simulink model "R"  (R2024a)
settings: Solver=VariableStepAuto  StartTime=0.0  StopTime=10*10^-6  RelTol=1e-3
undefined symbols (not defined in the file): c1, c3, rxDpIndex
libraries: commblkcod2 x64, commofdm x64, commdigbbndam3 x64, commsink2 x1, commseqgen3 x1
(part 2 of 3)

== system R/4K QAM/MSC13 WiFi Modulation29 ==
  In1 : Inport
  BCH Encoder : commblkcod2/BCH Encoder  n=47040  k=39200  specShortening=off  shortenedK=5  specGenPoly=off  genPoly='X^10 + X^8 + X^5 + X^4 + X^2 + X + 1'  specPrimPoly=off  prPoly='X^4 + X + 1'  specDisableGenCheck=off  specPuncture=off  punctVec=[ones(8,1); zeros(2,1)]
  OFDM Modulator : commofdm/OFDM Modulator  StatePerturbationForJacobian=1.0e-05  FFTLength=4096  NumGuardBandCarriers=[88; 88]  InsertDCNull=off  PilotInputPort=off  PilotCarrierIndices=[52;104;156;208;260]  CyclicPrefixLength=0  Windowing=off  WindowLength=1  OversamplingFactor=1  NumSymbols=1  NumTransmitAntennas=1  SimulateUsing=Interpreted execution
  Rectangular QAM Modulator Baseband : commdigbbndam3/Rectangular QAM Modulator Baseband  M=4096  InType=Bit  Enc=Gray  Mapping=[0:15]  PowType=Min. distance between symbols  MinDist=2  AvgPow=1  PeakPow=1  Ph=0  outDtype=double  outWordLen=16  outUDDataType=sfix(16)  outFracLenMode=Best precision  outFracLen=15  outDataTypeStr=double  outLastDataTypeStr=double
  Out1 : Outport
  wires:
  Rectangular QAM Modulator Baseband/1 -> OFDM Modulator/1
  OFDM Modulator/1 -> Out1/1
  BCH Encoder/1 -> Rectangular QAM Modulator Baseband/1
  In1/1 -> BCH Encoder/1

== system R/4K QAM/MSC13 WiFi Modulation3 ==
  In1 : Inport
  BCH Encoder : commblkcod2/BCH Encoder  n=47040  k=39200  specShortening=off  shortenedK=5  specGenPoly=off  genPoly='X^10 + X^8 + X^5 + X^4 + X^2 + X + 1'  specPrimPoly=off  prPoly='X^4 + X + 1'  specDisableGenCheck=off  specPuncture=off  punctVec=[ones(8,1); zeros(2,1)]
  OFDM Modulator : commofdm/OFDM Modulator  StatePerturbationForJacobian=1.0e-05  FFTLength=4096  NumGuardBandCarriers=[88; 88]  InsertDCNull=off  PilotInputPort=off  PilotCarrierIndices=[52;104;156;208;260]  CyclicPrefixLength=0  Windowing=off  WindowLength=1  OversamplingFactor=1  NumSymbols=1  NumTransmitAntennas=1  SimulateUsing=Interpreted execution
  Rectangular QAM Modulator Baseband : commdigbbndam3/Rectangular QAM Modulator Baseband  M=4096  InType=Bit  Enc=Gray  Mapping=[0:15]  PowType=Min. distance between symbols  MinDist=2  AvgPow=1  PeakPow=1  Ph=0  outDtype=double  outWordLen=16  outUDDataType=sfix(16)  outFracLenMode=Best precision  outFracLen=15  outDataTypeStr=double  outLastDataTypeStr=double
  Out1 : Outport
  wires:
  Rectangular QAM Modulator Baseband/1 -> OFDM Modulator/1
  OFDM Modulator/1 -> Out1/1
  BCH Encoder/1 -> Rectangular QAM Modulator Baseband/1
  In1/1 -> BCH Encoder/1

== system R/4K QAM/MSC13 WiFi Modulation30 ==
  In1 : Inport
  BCH Encoder : commblkcod2/BCH Encoder  n=47040  k=39200  specShortening=off  shortenedK=5  specGenPoly=off  genPoly='X^10 + X^8 + X^5 + X^4 + X^2 + X + 1'  specPrimPoly=off  prPoly='X^4 + X + 1'  specDisableGenCheck=off  specPuncture=off  punctVec=[ones(8,1); zeros(2,1)]
  OFDM Modulator : commofdm/OFDM Modulator  StatePerturbationForJacobian=1.0e-05  FFTLength=4096  NumGuardBandCarriers=[88; 88]  InsertDCNull=off  PilotInputPort=off  PilotCarrierIndices=[52;104;156;208;260]  CyclicPrefixLength=0  Windowing=off  WindowLength=1  OversamplingFactor=1  NumSymbols=1  NumTransmitAntennas=1  SimulateUsing=Interpreted execution
  Rectangular QAM Modulator Baseband : commdigbbndam3/Rectangular QAM Modulator Baseband  M=4096  InType=Bit  Enc=Gray  Mapping=[0:15]  PowType=Min. distance between symbols  MinDist=2  AvgPow=1  PeakPow=1  Ph=0  outDtype=double  outWordLen=16  outUDDataType=sfix(16)  outFracLenMode=Best precision  outFracLen=15  outDataTypeStr=double  outLastDataTypeStr=double
  Out1 : Outport
  wires:
  Rectangular QAM Modulator Baseband/1 -> OFDM Modulator/1
  OFDM Modulator/1 -> Out1/1
  BCH Encoder/1 -> Rectangular QAM Modulator Baseband/1
  In1/1 -> BCH Encoder/1

== system R/4K QAM/MSC13 WiFi Modulation31 ==
  In1 : Inport
  BCH Encoder : commblkcod2/BCH Encoder  n=47040  k=39200  specShortening=off  shortenedK=5  specGenPoly=off  genPoly='X^10 + X^8 + X^5 + X^4 + X^2 + X + 1'  specPrimPoly=off  prPoly='X^4 + X + 1'  specDisableGenCheck=off  specPuncture=off  punctVec=[ones(8,1); zeros(2,1)]
  OFDM Modulator : commofdm/OFDM Modulator  StatePerturbationForJacobian=1.0e-05  FFTLength=4096  NumGuardBandCarriers=[88; 88]  InsertDCNull=off  PilotInputPort=off  PilotCarrierIndices=[52;104;156;208;260]  CyclicPrefixLength=0  Windowing=off  WindowLength=1  OversamplingFactor=1  NumSymbols=1  NumTransmitAntennas=1  SimulateUsing=Interpreted execution
  Rectangular QAM Modulator Baseband : commdigbbndam3/Rectangular QAM Modulator Baseband  M=4096  InType=Bit  Enc=Gray  Mapping=[0:15]  PowType=Min. distance between symbols  MinDist=2  AvgPow=1  PeakPow=1  Ph=0  outDtype=double  outWordLen=16  outUDDataType=sfix(16)  outFracLenMode=Best precision  outFracLen=15  outDataTypeStr=double  outLastDataTypeStr=double
  Out1 : Outport
  wires:
  Rectangular QAM Modulator Baseband/1 -> OFDM Modulator/1
  OFDM Modulator/1 -> Out1/1
  BCH Encoder/1 -> Rectangular QAM Modulator Baseband/1
  In1/1 -> BCH Encoder/1

== system R/4K QAM/MSC13 WiFi Modulation4 ==
  In1 : Inport
  BCH Encoder : commblkcod2/BCH Encoder  n=47040  k=39200  specShortening=off  shortenedK=5  specGenPoly=off  genPoly='X^10 + X^8 + X^5 + X^4 + X^2 + X + 1'  specPrimPoly=off  prPoly='X^4 + X + 1'  specDisableGenCheck=off  specPuncture=off  punctVec=[ones(8,1); zeros(2,1)]
  OFDM Modulator : commofdm/OFDM Modulator  StatePerturbationForJacobian=1.0e-05  FFTLength=4096  NumGuardBandCarriers=[88; 88]  InsertDCNull=off  PilotInputPort=off  PilotCarrierIndices=[52;104;156;208;260]  CyclicPrefixLength=0  Windowing=off  WindowLength=1  OversamplingFactor=1  NumSymbols=1  NumTransmitAntennas=1  SimulateUsing=Interpreted execution
  Rectangular QAM Modulator Baseband : commdigbbndam3/Rectangular QAM Modulator Baseband  M=4096  InType=Bit  Enc=Gray  Mapping=[0:15]  PowType=Min. distance between symbols  MinDist=2  AvgPow=1  PeakPow=1  Ph=0  outDtype=double  outWordLen=16  outUDDataType=sfix(16)  outFracLenMode=Best precision  outFracLen=15  outDataTypeStr=double  outLastDataTypeStr=double
  Out1 : Outport
  wires:
  Rectangular QAM Modulator Baseband/1 -> OFDM Modulator/1
  OFDM Modulator/1 -> Out1/1
  BCH Encoder/1 -> Rectangular QAM Modulator Baseband/1
  In1/1 -> BCH Encoder/1

== system R/4K QAM/MSC13 WiFi Modulation5 ==
  In1 : Inport
  BCH Encoder : commblkcod2/BCH Encoder  n=47040  k=39200  specShortening=off  shortenedK=5  specGenPoly=off  genPoly='X^10 + X^8 + X^5 + X^4 + X^2 + X + 1'  specPrimPoly=off  prPoly='X^4 + X + 1'  specDisableGenCheck=off  specPuncture=off  punctVec=[ones(8,1); zeros(2,1)]
  OFDM Modulator : commofdm/OFDM Modulator  StatePerturbationForJacobian=1.0e-05  FFTLength=4096  NumGuardBandCarriers=[88; 88]  InsertDCNull=off  PilotInputPort=off  PilotCarrierIndices=[52;104;156;208;260]  CyclicPrefixLength=0  Windowing=off  WindowLength=1  OversamplingFactor=1  NumSymbols=1  NumTransmitAntennas=1  SimulateUsing=Interpreted execution
  Rectangular QAM Modulator Baseband : commdigbbndam3/Rectangular QAM Modulator Baseband  M=4096  InType=Bit  Enc=Gray  Mapping=[0:15]  PowType=Min. distance between symbols  MinDist=2  AvgPow=1  PeakPow=1  Ph=0  outDtype=double  outWordLen=16  outUDDataType=sfix(16)  outFracLenMode=Best precision  outFracLen=15  outDataTypeStr=double  outLastDataTypeStr=double
  Out1 : Outport
  wires:
  Rectangular QAM Modulator Baseband/1 -> OFDM Modulator/1
  OFDM Modulator/1 -> Out1/1
  BCH Encoder/1 -> Rectangular QAM Modulator Baseband/1
  In1/1 -> BCH Encoder/1

== system R/4K QAM/MSC13 WiFi Modulation6 ==
  In1 : Inport
  BCH Encoder : commblkcod2/BCH Encoder  n=47040  k=39200  specShortening=off  shortenedK=5  specGenPoly=off  genPoly='X^10 + X^8 + X^5 + X^4 + X^2 + X + 1'  specPrimPoly=off  prPoly='X^4 + X + 1'  specDisableGenCheck=off  specPuncture=off  punctVec=[ones(8,1); zeros(2,1)]
  OFDM Modulator : commofdm/OFDM Modulator  StatePerturbationForJacobian=1.0e-05  FFTLength=4096  NumGuardBandCarriers=[88; 88]  InsertDCNull=off  PilotInputPort=off  PilotCarrierIndices=[52;104;156;208;260]  CyclicPrefixLength=0  Windowing=off  WindowLength=1  OversamplingFactor=1  NumSymbols=1  NumTransmitAntennas=1  SimulateUsing=Interpreted execution
  Rectangular QAM Modulator Baseband : commdigbbndam3/Rectangular QAM Modulator Baseband  M=4096  InType=Bit  Enc=Gray  Mapping=[0:15]  PowType=Min. distance between symbols  MinDist=2  AvgPow=1  PeakPow=1  Ph=0  outDtype=double  outWordLen=16  outUDDataType=sfix(16)  outFracLenMode=Best precision  outFracLen=15  outDataTypeStr=double  outLastDataTypeStr=double
  Out1 : Outport
  wires:
  Rectangular QAM Modulator Baseband/1 -> OFDM Modulator/1
  OFDM Modulator/1 -> Out1/1
  BCH Encoder/1 -> Rectangular QAM Modulator Baseband/1
  In1/1 -> BCH Encoder/1

== system R/4K QAM/MSC13 WiFi Modulation7 ==
  In1 : Inport
  BCH Encoder : commblkcod2/BCH Encoder  n=47040  k=39200  specShortening=off  shortenedK=5  specGenPoly=off  genPoly='X^10 + X^8 + X^5 + X^4 + X^2 + X + 1'  specPrimPoly=off  prPoly='X^4 + X + 1'  specDisableGenCheck=off  specPuncture=off  punctVec=[ones(8,1); zeros(2,1)]
  OFDM Modulator : commofdm/OFDM Modulator  StatePerturbationForJacobian=1.0e-05  FFTLength=4096  NumGuardBandCarriers=[88; 88]  InsertDCNull=off  PilotInputPort=off  PilotCarrierIndices=[52;104;156;208;260]  CyclicPrefixLength=0  Windowing=off  WindowLength=1  OversamplingFactor=1  NumSymbols=1  NumTransmitAntennas=1  SimulateUsing=Interpreted execution
  Rectangular QAM Modulator Baseband : commdigbbndam3/Rectangular QAM Modulator Baseband  M=4096  InType=Bit  Enc=Gray  Mapping=[0:15]  PowType=Min. distance between symbols  MinDist=2  AvgPow=1  PeakPow=1  Ph=0  outDtype=double  outWordLen=16  outUDDataType=sfix(16)  outFracLenMode=Best precision  outFracLen=15  outDataTypeStr=double  outLastDataTypeStr=double
  Out1 : Outport
  wires:
  Rectangular QAM Modulator Baseband/1 -> OFDM Modulator/1
  OFDM Modulator/1 -> Out1/1
  BCH Encoder/1 -> Rectangular QAM Modulator Baseband/1
  In1/1 -> BCH Encoder/1

== system R/4K QAM/MSC13 WiFi Modulation8 ==
  In1 : Inport
  BCH Encoder : commblkcod2/BCH Encoder  n=47040  k=39200  specShortening=off  shortenedK=5  specGenPoly=off  genPoly='X^10 + X^8 + X^5 + X^4 + X^2 + X + 1'  specPrimPoly=off  prPoly='X^4 + X + 1'  specDisableGenCheck=off  specPuncture=off  punctVec=[ones(8,1); zeros(2,1)]
  OFDM Modulator : commofdm/OFDM Modulator  StatePerturbationForJacobian=1.0e-05  FFTLength=4096  NumGuardBandCarriers=[88; 88]  InsertDCNull=off  PilotInputPort=off  PilotCarrierIndices=[52;104;156;208;260]  CyclicPrefixLength=0  Windowing=off  WindowLength=1  OversamplingFactor=1  NumSymbols=1  NumTransmitAntennas=1  SimulateUsing=Interpreted execution
  Rectangular QAM Modulator Baseband : commdigbbndam3/Rectangular QAM Modulator Baseband  M=4096  InType=Bit  Enc=Gray  Mapping=[0:15]  PowType=Min. distance between symbols  MinDist=2  AvgPow=1  PeakPow=1  Ph=0  outDtype=double  outWordLen=16  outUDDataType=sfix(16)  outFracLenMode=Best precision  outFracLen=15  outDataTypeStr=double  outLastDataTypeStr=double
  Out1 : Outport
  wires:
  Rectangular QAM Modulator Baseband/1 -> OFDM Modulator/1
  OFDM Modulator/1 -> Out1/1
  BCH Encoder/1 -> Rectangular QAM Modulator Baseband/1
  In1/1 -> BCH Encoder/1

== system R/4K QAM/MSC13 WiFi Modulation9 ==
  In1 : Inport
  BCH Encoder : commblkcod2/BCH Encoder  n=47040  k=39200  specShortening=off  shortenedK=5  specGenPoly=off  genPoly='X^10 + X^8 + X^5 + X^4 + X^2 + X + 1'  specPrimPoly=off  prPoly='X^4 + X + 1'  specDisableGenCheck=off  specPuncture=off  punctVec=[ones(8,1); zeros(2,1)]
  OFDM Modulator : commofdm/OFDM Modulator  StatePerturbationForJacobian=1.0e-05  FFTLength=4096  NumGuardBandCarriers=[88; 88]  InsertDCNull=off  PilotInputPort=off  PilotCarrierIndices=[52;104;156;208;260]  CyclicPrefixLength=0  Windowing=off  WindowLength=1  OversamplingFactor=1  NumSymbols=1  NumTransmitAntennas=1  SimulateUsing=Interpreted execution
  Rectangular QAM Modulator Baseband : commdigbbndam3/Rectangular QAM Modulator Baseband  M=4096  InType=Bit  Enc=Gray  Mapping=[0:15]  PowType=Min. distance between symbols  MinDist=2  AvgPow=1  PeakPow=1  Ph=0  outDtype=double  outWordLen=16  outUDDataType=sfix(16)  outFracLenMode=Best precision  outFracLen=15  outDataTypeStr=double  outLastDataTypeStr=double
  Out1 : Outport
  wires:
  Rectangular QAM Modulator Baseband/1 -> OFDM Modulator/1
  OFDM Modulator/1 -> Out1/1
  BCH Encoder/1 -> Rectangular QAM Modulator Baseband/1
  In1/1 -> BCH Encoder/1

== system R/Subsystem1/MCS13 WiFi Demodulator1 ==
  In1 : Inport
  BCH Decoder1 : commblkcod2/BCH Decoder  n=47040  k=39200  specShortening=off  shortenedK=5  specGenPoly=off  genPoly='X^10 + X^8 + X^5 + X^4 + X^2 + X + 1'  specPrimPoly=off  prPoly='X^4 + X + 1'  specDisableGenCheck=off  specPuncture=off  punctVec=[ones(8,1); zeros(2,1)]  specErasurePort=off  showNumErr=off
  OFDM Demodulator1 : commofdm/OFDM Demodulator  StatePerturbationForJacobian=1.0e-05  FFTLength=4096  NumGuardBandCarriers=[88; 88]  RemoveDCCarrier=off  PilotOutputPort=off  PilotCarrierIndices=[35;60;85;110;135;160;185;210;235;260;285;310;335;360;385;410;435;460;485;510;535;560;585;610;635;660;685;710;735;760;785;810;835;860;885;910;935;960;985;1010;1035;1060;1085;1110;1135;1160;1185;1210;1235;1260;1285;1310;1335;1360;1385;1410;1435;1460;1485;1510;1535;1560;1585;1610;1635;1660;1685;1710;1735;1760;1785;1810;1835;1860;1885;1910;1935;1960;1985;2010;2035]  CyclicPrefixLength=0  OversamplingFactor=1  NumSymbols=1  NumReceiveAntennas=1  SimulateUsing=Interpreted execution
  Rectangular QAM Demodulator Baseband1 : commdigbbndam3/Rectangular QAM Demodulator Baseband  M=4096  OutType=Bit  DecType=Hard decision  VarSource=Dialog  Variance=1  Dec=Gray  Mapping=[0:15]  PowType=Min. distance between symbols  MinDist=2  AvgPow=1  PeakPow=1  Ph=0  outDtype1=Inherit via internal rule  outDtype2=Inherit via internal rule  derotateFactorWordLen=16  derotateFactorDataTypeStr=Inherit: Same word length as input  derotateFactorLastDataTypeStr=Inherit: Same word length as input  denormFactorWordLen=16  denormFactorDataTypeStr=Inherit: Same word length as input  denormFactorLastDataTypeStr=Inherit: Same word length as input  prodOutWordLen=32  prodOutOverflowMode=Wrap  prodOutRoundingMode=Floor  prodOutOvFlMode=off  prodOutOvFlModeLastStrValue=off  sumWordLen=32
      settings: LibrarySourceBlock=|
      | commhdldigbbndam/Rectangular QAM
      | Demodulator
      | Baseband
  Out1 : Outport
  wires:
  BCH Decoder1/1 -> Out1/1
  OFDM Demodulator1/1 -> Rectangular QAM Demodulator Baseband1/1
  In1/1 -> OFDM Demodulator1/1
  Rectangular QAM Demodulator Baseband1/1 -> BCH Decoder1/1

== system R/Subsystem1/MCS13 WiFi Demodulator10 ==
  In1 : Inport
  BCH Decoder1 : commblkcod2/BCH Decoder  n=47040  k=39200  specShortening=off  shortenedK=5  specGenPoly=off  genPoly='X^10 + X^8 + X^5 + X^4 + X^2 + X + 1'  specPrimPoly=off  prPoly='X^4 + X + 1'  specDisableGenCheck=off  specPuncture=off  punctVec=[ones(8,1); zeros(2,1)]  specErasurePort=off  showNumErr=off
  OFDM Demodulator1 : commofdm/OFDM Demodulator  StatePerturbationForJacobian=1.0e-05  FFTLength=4096  NumGuardBandCarriers=[88; 88]  RemoveDCCarrier=off  PilotOutputPort=off  PilotCarrierIndices=[35;60;85;110;135;160;185;210;235;260;285;310;335;360;385;410;435;460;485;510;535;560;585;610;635;660;685;710;735;760;785;810;835;860;885;910;935;960;985;1010;1035;1060;1085;1110;1135;1160;1185;1210;1235;1260;1285;1310;1335;1360;1385;1410;1435;1460;1485;1510;1535;1560;1585;1610;1635;1660;1685;1710;1735;1760;1785;1810;1835;1860;1885;1910;1935;1960;1985;2010;2035]  CyclicPrefixLength=0  OversamplingFactor=1  NumSymbols=1  NumReceiveAntennas=1  SimulateUsing=Interpreted execution
  Rectangular QAM Demodulator Baseband1 : commdigbbndam3/Rectangular QAM Demodulator Baseband  M=4096  OutType=Bit  DecType=Hard decision  VarSource=Dialog  Variance=1  Dec=Gray  Mapping=[0:15]  PowType=Min. distance between symbols  MinDist=2  AvgPow=1  PeakPow=1  Ph=0  outDtype1=Inherit via internal rule  outDtype2=Inherit via internal rule  derotateFactorWordLen=16  derotateFactorDataTypeStr=Inherit: Same word length as input  derotateFactorLastDataTypeStr=Inherit: Same word length as input  denormFactorWordLen=16  denormFactorDataTypeStr=Inherit: Same word length as input  denormFactorLastDataTypeStr=Inherit: Same word length as input  prodOutWordLen=32  prodOutOverflowMode=Wrap  prodOutRoundingMode=Floor  prodOutOvFlMode=off  prodOutOvFlModeLastStrValue=off  sumWordLen=32
      settings: LibrarySourceBlock=|
      | commhdldigbbndam/Rectangular QAM
      | Demodulator
      | Baseband
  Out1 : Outport
  wires:
  BCH Decoder1/1 -> Out1/1
  OFDM Demodulator1/1 -> Rectangular QAM Demodulator Baseband1/1
  In1/1 -> OFDM Demodulator1/1
  Rectangular QAM Demodulator Baseband1/1 -> BCH Decoder1/1

== system R/Subsystem1/MCS13 WiFi Demodulator11 ==
  In1 : Inport
  BCH Decoder1 : commblkcod2/BCH Decoder  n=47040  k=39200  specShortening=off  shortenedK=5  specGenPoly=off  genPoly='X^10 + X^8 + X^5 + X^4 + X^2 + X + 1'  specPrimPoly=off  prPoly='X^4 + X + 1'  specDisableGenCheck=off  specPuncture=off  punctVec=[ones(8,1); zeros(2,1)]  specErasurePort=off  showNumErr=off
  OFDM Demodulator1 : commofdm/OFDM Demodulator  StatePerturbationForJacobian=1.0e-05  FFTLength=4096  NumGuardBandCarriers=[88; 88]  RemoveDCCarrier=off  PilotOutputPort=off  PilotCarrierIndices=[35;60;85;110;135;160;185;210;235;260;285;310;335;360;385;410;435;460;485;510;535;560;585;610;635;660;685;710;735;760;785;810;835;860;885;910;935;960;985;1010;1035;1060;1085;1110;1135;1160;1185;1210;1235;1260;1285;1310;1335;1360;1385;1410;1435;1460;1485;1510;1535;1560;1585;1610;1635;1660;1685;1710;1735;1760;1785;1810;1835;1860;1885;1910;1935;1960;1985;2010;2035]  CyclicPrefixLength=0  OversamplingFactor=1  NumSymbols=1  NumReceiveAntennas=1  SimulateUsing=Interpreted execution
  Rectangular QAM Demodulator Baseband1 : commdigbbndam3/Rectangular QAM Demodulator Baseband  M=4096  OutType=Bit  DecType=Hard decision  VarSource=Dialog  Variance=1  Dec=Gray  Mapping=[0:15]  PowType=Min. distance between symbols  MinDist=2  AvgPow=1  PeakPow=1  Ph=0  outDtype1=Inherit via internal rule  outDtype2=Inherit via internal rule  derotateFactorWordLen=16  derotateFactorDataTypeStr=Inherit: Same word length as input  derotateFactorLastDataTypeStr=Inherit: Same word length as input  denormFactorWordLen=16  denormFactorDataTypeStr=Inherit: Same word length as input  denormFactorLastDataTypeStr=Inherit: Same word length as input  prodOutWordLen=32  prodOutOverflowMode=Wrap  prodOutRoundingMode=Floor  prodOutOvFlMode=off  prodOutOvFlModeLastStrValue=off  sumWordLen=32
      settings: LibrarySourceBlock=|
      | commhdldigbbndam/Rectangular QAM
      | Demodulator
      | Baseband
  Out1 : Outport
  wires:
  BCH Decoder1/1 -> Out1/1
  OFDM Demodulator1/1 -> Rectangular QAM Demodulator Baseband1/1
  In1/1 -> OFDM Demodulator1/1
  Rectangular QAM Demodulator Baseband1/1 -> BCH Decoder1/1

== system R/Subsystem1/MCS13 WiFi Demodulator12 ==
  In1 : Inport
  BCH Decoder1 : commblkcod2/BCH Decoder  n=47040  k=39200  specShortening=off  shortenedK=5  specGenPoly=off  genPoly='X^10 + X^8 + X^5 + X^4 + X^2 + X + 1'  specPrimPoly=off  prPoly='X^4 + X + 1'  specDisableGenCheck=off  specPuncture=off  punctVec=[ones(8,1); zeros(2,1)]  specErasurePort=off  showNumErr=off
  OFDM Demodulator1 : commofdm/OFDM Demodulator  StatePerturbationForJacobian=1.0e-05  FFTLength=4096  NumGuardBandCarriers=[88; 88]  RemoveDCCarrier=off  PilotOutputPort=off  PilotCarrierIndices=[35;60;85;110;135;160;185;210;235;260;285;310;335;360;385;410;435;460;485;510;535;560;585;610;635;660;685;710;735;760;785;810;835;860;885;910;935;960;985;1010;1035;1060;1085;1110;1135;1160;1185;1210;1235;1260;1285;1310;1335;1360;1385;1410;1435;1460;1485;1510;1535;1560;1585;1610;1635;1660;1685;1710;1735;1760;1785;1810;1835;1860;1885;1910;1935;1960;1985;2010;2035]  CyclicPrefixLength=0  OversamplingFactor=1  NumSymbols=1  NumReceiveAntennas=1  SimulateUsing=Interpreted execution
  Rectangular QAM Demodulator Baseband1 : commdigbbndam3/Rectangular QAM Demodulator Baseband  M=4096  OutType=Bit  DecType=Hard decision  VarSource=Dialog  Variance=1  Dec=Gray  Mapping=[0:15]  PowType=Min. distance between symbols  MinDist=2  AvgPow=1  PeakPow=1  Ph=0  outDtype1=Inherit via internal rule  outDtype2=Inherit via internal rule  derotateFactorWordLen=16  derotateFactorDataTypeStr=Inherit: Same word length as input  derotateFactorLastDataTypeStr=Inherit: Same word length as input  denormFactorWordLen=16  denormFactorDataTypeStr=Inherit: Same word length as input  denormFactorLastDataTypeStr=Inherit: Same word length as input  prodOutWordLen=32  prodOutOverflowMode=Wrap  prodOutRoundingMode=Floor  prodOutOvFlMode=off  prodOutOvFlModeLastStrValue=off  sumWordLen=32
      settings: LibrarySourceBlock=|
      | commhdldigbbndam/Rectangular QAM
      | Demodulator
      | Baseband
  Out1 : Outport
  wires:
  BCH Decoder1/1 -> Out1/1
  OFDM Demodulator1/1 -> Rectangular QAM Demodulator Baseband1/1
  In1/1 -> OFDM Demodulator1/1
  Rectangular QAM Demodulator Baseband1/1 -> BCH Decoder1/1

== system R/Subsystem1/MCS13 WiFi Demodulator13 ==
  In1 : Inport
  BCH Decoder1 : commblkcod2/BCH Decoder  n=47040  k=39200  specShortening=off  shortenedK=5  specGenPoly=off  genPoly='X^10 + X^8 + X^5 + X^4 + X^2 + X + 1'  specPrimPoly=off  prPoly='X^4 + X + 1'  specDisableGenCheck=off  specPuncture=off  punctVec=[ones(8,1); zeros(2,1)]  specErasurePort=off  showNumErr=off
  OFDM Demodulator1 : commofdm/OFDM Demodulator  StatePerturbationForJacobian=1.0e-05  FFTLength=4096  NumGuardBandCarriers=[88; 88]  RemoveDCCarrier=off  PilotOutputPort=off  PilotCarrierIndices=[35;60;85;110;135;160;185;210;235;260;285;310;335;360;385;410;435;460;485;510;535;560;585;610;635;660;685;710;735;760;785;810;835;860;885;910;935;960;985;1010;1035;1060;1085;1110;1135;1160;1185;1210;1235;1260;1285;1310;1335;1360;1385;1410;1435;1460;1485;1510;1535;1560;1585;1610;1635;1660;1685;1710;1735;1760;1785;1810;1835;1860;1885;1910;1935;1960;1985;2010;2035]  CyclicPrefixLength=0  OversamplingFactor=1  NumSymbols=1  NumReceiveAntennas=1  SimulateUsing=Interpreted execution
  Rectangular QAM Demodulator Baseband1 : commdigbbndam3/Rectangular QAM Demodulator Baseband  M=4096  OutType=Bit  DecType=Hard decision  VarSource=Dialog  Variance=1  Dec=Gray  Mapping=[0:15]  PowType=Min. distance between symbols  MinDist=2  AvgPow=1  PeakPow=1  Ph=0  outDtype1=Inherit via internal rule  outDtype2=Inherit via internal rule  derotateFactorWordLen=16  derotateFactorDataTypeStr=Inherit: Same word length as input  derotateFactorLastDataTypeStr=Inherit: Same word length as input  denormFactorWordLen=16  denormFactorDataTypeStr=Inherit: Same word length as input  denormFactorLastDataTypeStr=Inherit: Same word length as input  prodOutWordLen=32  prodOutOverflowMode=Wrap  prodOutRoundingMode=Floor  prodOutOvFlMode=off  prodOutOvFlModeLastStrValue=off  sumWordLen=32
      settings: LibrarySourceBlock=|
      | commhdldigbbndam/Rectangular QAM
      | Demodulator
      | Baseband
  Out1 : Outport
  wires:
  BCH Decoder1/1 -> Out1/1
  OFDM Demodulator1/1 -> Rectangular QAM Demodulator Baseband1/1
  In1/1 -> OFDM Demodulator1/1
  Rectangular QAM Demodulator Baseband1/1 -> BCH Decoder1/1

== system R/Subsystem1/MCS13 WiFi Demodulator14 ==
  In1 : Inport
  BCH Decoder1 : commblkcod2/BCH Decoder  n=47040  k=39200  specShortening=off  shortenedK=5  specGenPoly=off  genPoly='X^10 + X^8 + X^5 + X^4 + X^2 + X + 1'  specPrimPoly=off  prPoly='X^4 + X + 1'  specDisableGenCheck=off  specPuncture=off  punctVec=[ones(8,1); zeros(2,1)]  specErasurePort=off  showNumErr=off
  OFDM Demodulator1 : commofdm/OFDM Demodulator  StatePerturbationForJacobian=1.0e-05  FFTLength=4096  NumGuardBandCarriers=[88; 88]  RemoveDCCarrier=off  PilotOutputPort=off  PilotCarrierIndices=[35;60;85;110;135;160;185;210;235;260;285;310;335;360;385;410;435;460;485;510;535;560;585;610;635;660;685;710;735;760;785;810;835;860;885;910;935;960;985;1010;1035;1060;1085;1110;1135;1160;1185;1210;1235;1260;1285;1310;1335;1360;1385;1410;1435;1460;1485;1510;1535;1560;1585;1610;1635;1660;1685;1710;1735;1760;1785;1810;1835;1860;1885;1910;1935;1960;1985;2010;2035]  CyclicPrefixLength=0  OversamplingFactor=1  NumSymbols=1  NumReceiveAntennas=1  SimulateUsing=Interpreted execution
  Rectangular QAM Demodulator Baseband1 : commdigbbndam3/Rectangular QAM Demodulator Baseband  M=4096  OutType=Bit  DecType=Hard decision  VarSource=Dialog  Variance=1  Dec=Gray  Mapping=[0:15]  PowType=Min. distance between symbols  MinDist=2  AvgPow=1  PeakPow=1  Ph=0  outDtype1=Inherit via internal rule  outDtype2=Inherit via internal rule  derotateFactorWordLen=16  derotateFactorDataTypeStr=Inherit: Same word length as input  derotateFactorLastDataTypeStr=Inherit: Same word length as input  denormFactorWordLen=16  denormFactorDataTypeStr=Inherit: Same word length as input  denormFactorLastDataTypeStr=Inherit: Same word length as input  prodOutWordLen=32  prodOutOverflowMode=Wrap  prodOutRoundingMode=Floor  prodOutOvFlMode=off  prodOutOvFlModeLastStrValue=off  sumWordLen=32
      settings: LibrarySourceBlock=|
      | commhdldigbbndam/Rectangular QAM
      | Demodulator
      | Baseband
  Out1 : Outport
  wires:
  BCH Decoder1/1 -> Out1/1
  OFDM Demodulator1/1 -> Rectangular QAM Demodulator Baseband1/1
  In1/1 -> OFDM Demodulator1/1
  Rectangular QAM Demodulator Baseband1/1 -> BCH Decoder1/1

== system R/Subsystem1/MCS13 WiFi Demodulator15 ==
  In1 : Inport
  BCH Decoder1 : commblkcod2/BCH Decoder  n=47040  k=39200  specShortening=off  shortenedK=5  specGenPoly=off  genPoly='X^10 + X^8 + X^5 + X^4 + X^2 + X + 1'  specPrimPoly=off  prPoly='X^4 + X + 1'  specDisableGenCheck=off  specPuncture=off  punctVec=[ones(8,1); zeros(2,1)]  specErasurePort=off  showNumErr=off
  OFDM Demodulator1 : commofdm/OFDM Demodulator  StatePerturbationForJacobian=1.0e-05  FFTLength=4096  NumGuardBandCarriers=[88; 88]  RemoveDCCarrier=off  PilotOutputPort=off  PilotCarrierIndices=[35;60;85;110;135;160;185;210;235;260;285;310;335;360;385;410;435;460;485;510;535;560;585;610;635;660;685;710;735;760;785;810;835;860;885;910;935;960;985;1010;1035;1060;1085;1110;1135;1160;1185;1210;1235;1260;1285;1310;1335;1360;1385;1410;1435;1460;1485;1510;1535;1560;1585;1610;1635;1660;1685;1710;1735;1760;1785;1810;1835;1860;1885;1910;1935;1960;1985;2010;2035]  CyclicPrefixLength=0  OversamplingFactor=1  NumSymbols=1  NumReceiveAntennas=1  SimulateUsing=Interpreted execution
  Rectangular QAM Demodulator Baseband1 : commdigbbndam3/Rectangular QAM Demodulator Baseband  M=4096  OutType=Bit  DecType=Hard decision  VarSource=Dialog  Variance=1  Dec=Gray  Mapping=[0:15]  PowType=Min. distance between symbols  MinDist=2  AvgPow=1  PeakPow=1  Ph=0  outDtype1=Inherit via internal rule  outDtype2=Inherit via internal rule  derotateFactorWordLen=16  derotateFactorDataTypeStr=Inherit: Same word length as input  derotateFactorLastDataTypeStr=Inherit: Same word length as input  denormFactorWordLen=16  denormFactorDataTypeStr=Inherit: Same word length as input  denormFactorLastDataTypeStr=Inherit: Same word length as input  prodOutWordLen=32  prodOutOverflowMode=Wrap  prodOutRoundingMode=Floor  prodOutOvFlMode=off  prodOutOvFlModeLastStrValue=off  sumWordLen=32
      settings: LibrarySourceBlock=|
      | commhdldigbbndam/Rectangular QAM
      | Demodulator
      | Baseband
  Out1 : Outport
  wires:
  BCH Decoder1/1 -> Out1/1
  OFDM Demodulator1/1 -> Rectangular QAM Demodulator Baseband1/1
  In1/1 -> OFDM Demodulator1/1
  Rectangular QAM Demodulator Baseband1/1 -> BCH Decoder1/1

== system R/Subsystem1/MCS13 WiFi Demodulator16 ==
  In1 : Inport
  BCH Decoder1 : commblkcod2/BCH Decoder  n=47040  k=39200  specShortening=off  shortenedK=5  specGenPoly=off  genPoly='X^10 + X^8 + X^5 + X^4 + X^2 + X + 1'  specPrimPoly=off  prPoly='X^4 + X + 1'  specDisableGenCheck=off  specPuncture=off  punctVec=[ones(8,1); zeros(2,1)]  specErasurePort=off  showNumErr=off
  OFDM Demodulator1 : commofdm/OFDM Demodulator  StatePerturbationForJacobian=1.0e-05  FFTLength=4096  NumGuardBandCarriers=[88; 88]  RemoveDCCarrier=off  PilotOutputPort=off  PilotCarrierIndices=[35;60;85;110;135;160;185;210;235;260;285;310;335;360;385;410;435;460;485;510;535;560;585;610;635;660;685;710;735;760;785;810;835;860;885;910;935;960;985;1010;1035;1060;1085;1110;1135;1160;1185;1210;1235;1260;1285;1310;1335;1360;1385;1410;1435;1460;1485;1510;1535;1560;1585;1610;1635;1660;1685;1710;1735;1760;1785;1810;1835;1860;1885;1910;1935;1960;1985;2010;2035]  CyclicPrefixLength=0  OversamplingFactor=1  NumSymbols=1  NumReceiveAntennas=1  SimulateUsing=Interpreted execution
  Rectangular QAM Demodulator Baseband1 : commdigbbndam3/Rectangular QAM Demodulator Baseband  M=4096  OutType=Bit  DecType=Hard decision  VarSource=Dialog  Variance=1  Dec=Gray  Mapping=[0:15]  PowType=Min. distance between symbols  MinDist=2  AvgPow=1  PeakPow=1  Ph=0  outDtype1=Inherit via internal rule  outDtype2=Inherit via internal rule  derotateFactorWordLen=16  derotateFactorDataTypeStr=Inherit: Same word length as input  derotateFactorLastDataTypeStr=Inherit: Same word length as input  denormFactorWordLen=16  denormFactorDataTypeStr=Inherit: Same word length as input  denormFactorLastDataTypeStr=Inherit: Same word length as input  prodOutWordLen=32  prodOutOverflowMode=Wrap  prodOutRoundingMode=Floor  prodOutOvFlMode=off  prodOutOvFlModeLastStrValue=off  sumWordLen=32
      settings: LibrarySourceBlock=|
      | commhdldigbbndam/Rectangular QAM
      | Demodulator
      | Baseband
  Out1 : Outport
  wires:
  BCH Decoder1/1 -> Out1/1
  OFDM Demodulator1/1 -> Rectangular QAM Demodulator Baseband1/1
  In1/1 -> OFDM Demodulator1/1
  Rectangular QAM Demodulator Baseband1/1 -> BCH Decoder1/1

== system R/Subsystem1/MCS13 WiFi Demodulator17 ==
  In1 : Inport
  BCH Decoder1 : commblkcod2/BCH Decoder  n=47040  k=39200  specShortening=off  shortenedK=5  specGenPoly=off  genPoly='X^10 + X^8 + X^5 + X^4 + X^2 + X + 1'  specPrimPoly=off  prPoly='X^4 + X + 1'  specDisableGenCheck=off  specPuncture=off  punctVec=[ones(8,1); zeros(2,1)]  specErasurePort=off  showNumErr=off
  OFDM Demodulator1 : commofdm/OFDM Demodulator  StatePerturbationForJacobian=1.0e-05  FFTLength=4096  NumGuardBandCarriers=[88; 88]  RemoveDCCarrier=off  PilotOutputPort=off  PilotCarrierIndices=[35;60;85;110;135;160;185;210;235;260;285;310;335;360;385;410;435;460;485;510;535;560;585;610;635;660;685;710;735;760;785;810;835;860;885;910;935;960;985;1010;1035;1060;1085;1110;1135;1160;1185;1210;1235;1260;1285;1310;1335;1360;1385;1410;1435;1460;1485;1510;1535;1560;1585;1610;1635;1660;1685;1710;1735;1760;1785;1810;1835;1860;1885;1910;1935;1960;1985;2010;2035]  CyclicPrefixLength=0  OversamplingFactor=1  NumSymbols=1  NumReceiveAntennas=1  SimulateUsing=Interpreted execution
  Rectangular QAM Demodulator Baseband1 : commdigbbndam3/Rectangular QAM Demodulator Baseband  M=4096  OutType=Bit  DecType=Hard decision  VarSource=Dialog  Variance=1  Dec=Gray  Mapping=[0:15]  PowType=Min. distance between symbols  MinDist=2  AvgPow=1  PeakPow=1  Ph=0  outDtype1=Inherit via internal rule  outDtype2=Inherit via internal rule  derotateFactorWordLen=16  derotateFactorDataTypeStr=Inherit: Same word length as input  derotateFactorLastDataTypeStr=Inherit: Same word length as input  denormFactorWordLen=16  denormFactorDataTypeStr=Inherit: Same word length as input  denormFactorLastDataTypeStr=Inherit: Same word length as input  prodOutWordLen=32  prodOutOverflowMode=Wrap  prodOutRoundingMode=Floor  prodOutOvFlMode=off  prodOutOvFlModeLastStrValue=off  sumWordLen=32
      settings: LibrarySourceBlock=|
      | commhdldigbbndam/Rectangular QAM
      | Demodulator
      | Baseband
  Out1 : Outport
  wires:
  BCH Decoder1/1 -> Out1/1
  OFDM Demodulator1/1 -> Rectangular QAM Demodulator Baseband1/1
  In1/1 -> OFDM Demodulator1/1
  Rectangular QAM Demodulator Baseband1/1 -> BCH Decoder1/1

== system R/Subsystem1/MCS13 WiFi Demodulator18 ==
  In1 : Inport
  BCH Decoder1 : commblkcod2/BCH Decoder  n=47040  k=39200  specShortening=off  shortenedK=5  specGenPoly=off  genPoly='X^10 + X^8 + X^5 + X^4 + X^2 + X + 1'  specPrimPoly=off  prPoly='X^4 + X + 1'  specDisableGenCheck=off  specPuncture=off  punctVec=[ones(8,1); zeros(2,1)]  specErasurePort=off  showNumErr=off
  OFDM Demodulator1 : commofdm/OFDM Demodulator  StatePerturbationForJacobian=1.0e-05  FFTLength=4096  NumGuardBandCarriers=[88; 88]  RemoveDCCarrier=off  PilotOutputPort=off  PilotCarrierIndices=[35;60;85;110;135;160;185;210;235;260;285;310;335;360;385;410;435;460;485;510;535;560;585;610;635;660;685;710;735;760;785;810;835;860;885;910;935;960;985;1010;1035;1060;1085;1110;1135;1160;1185;1210;1235;1260;1285;1310;1335;1360;1385;1410;1435;1460;1485;1510;1535;1560;1585;1610;1635;1660;1685;1710;1735;1760;1785;1810;1835;1860;1885;1910;1935;1960;1985;2010;2035]  CyclicPrefixLength=0  OversamplingFactor=1  NumSymbols=1  NumReceiveAntennas=1  SimulateUsing=Interpreted execution
  Rectangular QAM Demodulator Baseband1 : commdigbbndam3/Rectangular QAM Demodulator Baseband  M=4096  OutType=Bit  DecType=Hard decision  VarSource=Dialog  Variance=1  Dec=Gray  Mapping=[0:15]  PowType=Min. distance between symbols  MinDist=2  AvgPow=1  PeakPow=1  Ph=0  outDtype1=Inherit via internal rule  outDtype2=Inherit via internal rule  derotateFactorWordLen=16  derotateFactorDataTypeStr=Inherit: Same word length as input  derotateFactorLastDataTypeStr=Inherit: Same word length as input  denormFactorWordLen=16  denormFactorDataTypeStr=Inherit: Same word length as input  denormFactorLastDataTypeStr=Inherit: Same word length as input  prodOutWordLen=32  prodOutOverflowMode=Wrap  prodOutRoundingMode=Floor  prodOutOvFlMode=off  prodOutOvFlModeLastStrValue=off  sumWordLen=32
      settings: LibrarySourceBlock=|
      | commhdldigbbndam/Rectangular QAM
      | Demodulator
      | Baseband
  Out1 : Outport
  wires:
  BCH Decoder1/1 -> Out1/1
  OFDM Demodulator1/1 -> Rectangular QAM Demodulator Baseband1/1
  In1/1 -> OFDM Demodulator1/1
  Rectangular QAM Demodulator Baseband1/1 -> BCH Decoder1/1

== system R/Subsystem1/MCS13 WiFi Demodulator19 ==
  In1 : Inport
  BCH Decoder1 : commblkcod2/BCH Decoder  n=47040  k=39200  specShortening=off  shortenedK=5  specGenPoly=off  genPoly='X^10 + X^8 + X^5 + X^4 + X^2 + X + 1'  specPrimPoly=off  prPoly='X^4 + X + 1'  specDisableGenCheck=off  specPuncture=off  punctVec=[ones(8,1); zeros(2,1)]  specErasurePort=off  showNumErr=off
  OFDM Demodulator1 : commofdm/OFDM Demodulator  StatePerturbationForJacobian=1.0e-05  FFTLength=4096  NumGuardBandCarriers=[88; 88]  RemoveDCCarrier=off  PilotOutputPort=off  PilotCarrierIndices=[35;60;85;110;135;160;185;210;235;260;285;310;335;360;385;410;435;460;485;510;535;560;585;610;635;660;685;710;735;760;785;810;835;860;885;910;935;960;985;1010;1035;1060;1085;1110;1135;1160;1185;1210;1235;1260;1285;1310;1335;1360;1385;1410;1435;1460;1485;1510;1535;1560;1585;1610;1635;1660;1685;1710;1735;1760;1785;1810;1835;1860;1885;1910;1935;1960;1985;2010;2035]  CyclicPrefixLength=0  OversamplingFactor=1  NumSymbols=1  NumReceiveAntennas=1  SimulateUsing=Interpreted execution
  Rectangular QAM Demodulator Baseband1 : commdigbbndam3/Rectangular QAM Demodulator Baseband  M=4096  OutType=Bit  DecType=Hard decision  VarSource=Dialog  Variance=1  Dec=Gray  Mapping=[0:15]  PowType=Min. distance between symbols  MinDist=2  AvgPow=1  PeakPow=1  Ph=0  outDtype1=Inherit via internal rule  outDtype2=Inherit via internal rule  derotateFactorWordLen=16  derotateFactorDataTypeStr=Inherit: Same word length as input  derotateFactorLastDataTypeStr=Inherit: Same word length as input  denormFactorWordLen=16  denormFactorDataTypeStr=Inherit: Same word length as input  denormFactorLastDataTypeStr=Inherit: Same word length as input  prodOutWordLen=32  prodOutOverflowMode=Wrap  prodOutRoundingMode=Floor  prodOutOvFlMode=off  prodOutOvFlModeLastStrValue=off  sumWordLen=32
      settings: LibrarySourceBlock=|
      | commhdldigbbndam/Rectangular QAM
      | Demodulator
      | Baseband
  Out1 : Outport
  wires:
  BCH Decoder1/1 -> Out1/1
  OFDM Demodulator1/1 -> Rectangular QAM Demodulator Baseband1/1
  In1/1 -> OFDM Demodulator1/1
  Rectangular QAM Demodulator Baseband1/1 -> BCH Decoder1/1

== system R/Subsystem1/MCS13 WiFi Demodulator2 ==
  In1 : Inport
  BCH Decoder1 : commblkcod2/BCH Decoder  n=47040  k=39200  specShortening=off  shortenedK=5  specGenPoly=off  genPoly='X^10 + X^8 + X^5 + X^4 + X^2 + X + 1'  specPrimPoly=off  prPoly='X^4 + X + 1'  specDisableGenCheck=off  specPuncture=off  punctVec=[ones(8,1); zeros(2,1)]  specErasurePort=off  showNumErr=off
  OFDM Demodulator1 : commofdm/OFDM Demodulator  StatePerturbationForJacobian=1.0e-05  FFTLength=4096  NumGuardBandCarriers=[88; 88]  RemoveDCCarrier=off  PilotOutputPort=off  PilotCarrierIndices=[35;60;85;110;135;160;185;210;235;260;285;310;335;360;385;410;435;460;485;510;535;560;585;610;635;660;685;710;735;760;785;810;835;860;885;910;935;960;985;1010;1035;1060;1085;1110;1135;1160;1185;1210;1235;1260;1285;1310;1335;1360;1385;1410;1435;1460;1485;1510;1535;1560;1585;1610;1635;1660;1685;1710;1735;1760;1785;1810;1835;1860;1885;1910;1935;1960;1985;2010;2035]  CyclicPrefixLength=0  OversamplingFactor=1  NumSymbols=1  NumReceiveAntennas=1  SimulateUsing=Interpreted execution
  Rectangular QAM Demodulator Baseband1 : commdigbbndam3/Rectangular QAM Demodulator Baseband  M=4096  OutType=Bit  DecType=Hard decision  VarSource=Dialog  Variance=1  Dec=Gray  Mapping=[0:15]  PowType=Min. distance between symbols  MinDist=2  AvgPow=1  PeakPow=1  Ph=0  outDtype1=Inherit via internal rule  outDtype2=Inherit via internal rule  derotateFactorWordLen=16  derotateFactorDataTypeStr=Inherit: Same word length as input  derotateFactorLastDataTypeStr=Inherit: Same word length as input  denormFactorWordLen=16  denormFactorDataTypeStr=Inherit: Same word length as input  denormFactorLastDataTypeStr=Inherit: Same word length as input  prodOutWordLen=32  prodOutOverflowMode=Wrap  prodOutRoundingMode=Floor  prodOutOvFlMode=off  prodOutOvFlModeLastStrValue=off  sumWordLen=32
      settings: LibrarySourceBlock=|
      | commhdldigbbndam/Rectangular QAM
      | Demodulator
      | Baseband
  Out1 : Outport
  wires:
  BCH Decoder1/1 -> Out1/1
  OFDM Demodulator1/1 -> Rectangular QAM Demodulator Baseband1/1
  In1/1 -> OFDM Demodulator1/1
  Rectangular QAM Demodulator Baseband1/1 -> BCH Decoder1/1

== system R/Subsystem1/MCS13 WiFi Demodulator20 ==
  In1 : Inport
  BCH Decoder1 : commblkcod2/BCH Decoder  n=47040  k=39200  specShortening=off  shortenedK=5  specGenPoly=off  genPoly='X^10 + X^8 + X^5 + X^4 + X^2 + X + 1'  specPrimPoly=off  prPoly='X^4 + X + 1'  specDisableGenCheck=off  specPuncture=off  punctVec=[ones(8,1); zeros(2,1)]  specErasurePort=off  showNumErr=off
  OFDM Demodulator1 : commofdm/OFDM Demodulator  StatePerturbationForJacobian=1.0e-05  FFTLength=4096  NumGuardBandCarriers=[88; 88]  RemoveDCCarrier=off  PilotOutputPort=off  PilotCarrierIndices=[35;60;85;110;135;160;185;210;235;260;285;310;335;360;385;410;435;460;485;510;535;560;585;610;635;660;685;710;735;760;785;810;835;860;885;910;935;960;985;1010;1035;1060;1085;1110;1135;1160;1185;1210;1235;1260;1285;1310;1335;1360;1385;1410;1435;1460;1485;1510;1535;1560;1585;1610;1635;1660;1685;1710;1735;1760;1785;1810;1835;1860;1885;1910;1935;1960;1985;2010;2035]  CyclicPrefixLength=0  OversamplingFactor=1  NumSymbols=1  NumReceiveAntennas=1  SimulateUsing=Interpreted execution
  Rectangular QAM Demodulator Baseband1 : commdigbbndam3/Rectangular QAM Demodulator Baseband  M=4096  OutType=Bit  DecType=Hard decision  VarSource=Dialog  Variance=1  Dec=Gray  Mapping=[0:15]  PowType=Min. distance between symbols  MinDist=2  AvgPow=1  PeakPow=1  Ph=0  outDtype1=Inherit via internal rule  outDtype2=Inherit via internal rule  derotateFactorWordLen=16  derotateFactorDataTypeStr=Inherit: Same word length as input  derotateFactorLastDataTypeStr=Inherit: Same word length as input  denormFactorWordLen=16  denormFactorDataTypeStr=Inherit: Same word length as input  denormFactorLastDataTypeStr=Inherit: Same word length as input  prodOutWordLen=32  prodOutOverflowMode=Wrap  prodOutRoundingMode=Floor  prodOutOvFlMode=off  prodOutOvFlModeLastStrValue=off  sumWordLen=32
      settings: LibrarySourceBlock=|
      | commhdldigbbndam/Rectangular QAM
      | Demodulator
      | Baseband
  Out1 : Outport
  wires:
  BCH Decoder1/1 -> Out1/1
  OFDM Demodulator1/1 -> Rectangular QAM Demodulator Baseband1/1
  In1/1 -> OFDM Demodulator1/1
  Rectangular QAM Demodulator Baseband1/1 -> BCH Decoder1/1

== system R/Subsystem1/MCS13 WiFi Demodulator21 ==
  In1 : Inport
  BCH Decoder1 : commblkcod2/BCH Decoder  n=47040  k=39200  specShortening=off  shortenedK=5  specGenPoly=off  genPoly='X^10 + X^8 + X^5 + X^4 + X^2 + X + 1'  specPrimPoly=off  prPoly='X^4 + X + 1'  specDisableGenCheck=off  specPuncture=off  punctVec=[ones(8,1); zeros(2,1)]  specErasurePort=off  showNumErr=off
  OFDM Demodulator1 : commofdm/OFDM Demodulator  StatePerturbationForJacobian=1.0e-05  FFTLength=4096  NumGuardBandCarriers=[88; 88]  RemoveDCCarrier=off  PilotOutputPort=off  PilotCarrierIndices=[35;60;85;110;135;160;185;210;235;260;285;310;335;360;385;410;435;460;485;510;535;560;585;610;635;660;685;710;735;760;785;810;835;860;885;910;935;960;985;1010;1035;1060;1085;1110;1135;1160;1185;1210;1235;1260;1285;1310;1335;1360;1385;1410;1435;1460;1485;1510;1535;1560;1585;1610;1635;1660;1685;1710;1735;1760;1785;1810;1835;1860;1885;1910;1935;1960;1985;2010;2035]  CyclicPrefixLength=0  OversamplingFactor=1  NumSymbols=1  NumReceiveAntennas=1  SimulateUsing=Interpreted execution
  Rectangular QAM Demodulator Baseband1 : commdigbbndam3/Rectangular QAM Demodulator Baseband  M=4096  OutType=Bit  DecType=Hard decision  VarSource=Dialog  Variance=1  Dec=Gray  Mapping=[0:15]  PowType=Min. distance between symbols  MinDist=2  AvgPow=1  PeakPow=1  Ph=0  outDtype1=Inherit via internal rule  outDtype2=Inherit via internal rule  derotateFactorWordLen=16  derotateFactorDataTypeStr=Inherit: Same word length as input  derotateFactorLastDataTypeStr=Inherit: Same word length as input  denormFactorWordLen=16  denormFactorDataTypeStr=Inherit: Same word length as input  denormFactorLastDataTypeStr=Inherit: Same word length as input  prodOutWordLen=32  prodOutOverflowMode=Wrap  prodOutRoundingMode=Floor  prodOutOvFlMode=off  prodOutOvFlModeLastStrValue=off  sumWordLen=32
      settings: LibrarySourceBlock=|
      | commhdldigbbndam/Rectangular QAM
      | Demodulator
      | Baseband
  Out1 : Outport
  wires:
  BCH Decoder1/1 -> Out1/1
  OFDM Demodulator1/1 -> Rectangular QAM Demodulator Baseband1/1
  In1/1 -> OFDM Demodulator1/1
  Rectangular QAM Demodulator Baseband1/1 -> BCH Decoder1/1

== system R/Subsystem1/MCS13 WiFi Demodulator22 ==
  In1 : Inport
  BCH Decoder1 : commblkcod2/BCH Decoder  n=47040  k=39200  specShortening=off  shortenedK=5  specGenPoly=off  genPoly='X^10 + X^8 + X^5 + X^4 + X^2 + X + 1'  specPrimPoly=off  prPoly='X^4 + X + 1'  specDisableGenCheck=off  specPuncture=off  punctVec=[ones(8,1); zeros(2,1)]  specErasurePort=off  showNumErr=off
  OFDM Demodulator1 : commofdm/OFDM Demodulator  StatePerturbationForJacobian=1.0e-05  FFTLength=4096  NumGuardBandCarriers=[88; 88]  RemoveDCCarrier=off  PilotOutputPort=off  PilotCarrierIndices=[35;60;85;110;135;160;185;210;235;260;285;310;335;360;385;410;435;460;485;510;535;560;585;610;635;660;685;710;735;760;785;810;835;860;885;910;935;960;985;1010;1035;1060;1085;1110;1135;1160;1185;1210;1235;1260;1285;1310;1335;1360;1385;1410;1435;1460;1485;1510;1535;1560;1585;1610;1635;1660;1685;1710;1735;1760;1785;1810;1835;1860;1885;1910;1935;1960;1985;2010;2035]  CyclicPrefixLength=0  OversamplingFactor=1  NumSymbols=1  NumReceiveAntennas=1  SimulateUsing=Interpreted execution
  Rectangular QAM Demodulator Baseband1 : commdigbbndam3/Rectangular QAM Demodulator Baseband  M=4096  OutType=Bit  DecType=Hard decision  VarSource=Dialog  Variance=1  Dec=Gray  Mapping=[0:15]  PowType=Min. distance between symbols  MinDist=2  AvgPow=1  PeakPow=1  Ph=0  outDtype1=Inherit via internal rule  outDtype2=Inherit via internal rule  derotateFactorWordLen=16  derotateFactorDataTypeStr=Inherit: Same word length as input  derotateFactorLastDataTypeStr=Inherit: Same word length as input  denormFactorWordLen=16  denormFactorDataTypeStr=Inherit: Same word length as input  denormFactorLastDataTypeStr=Inherit: Same word length as input  prodOutWordLen=32  prodOutOverflowMode=Wrap  prodOutRoundingMode=Floor  prodOutOvFlMode=off  prodOutOvFlModeLastStrValue=off  sumWordLen=32
      settings: LibrarySourceBlock=|
      | commhdldigbbndam/Rectangular QAM
      | Demodulator
      | Baseband
  Out1 : Outport
  wires:
  BCH Decoder1/1 -> Out1/1
  OFDM Demodulator1/1 -> Rectangular QAM Demodulator Baseband1/1
  In1/1 -> OFDM Demodulator1/1
  Rectangular QAM Demodulator Baseband1/1 -> BCH Decoder1/1

== system R/Subsystem1/MCS13 WiFi Demodulator23 ==
  In1 : Inport
  BCH Decoder1 : commblkcod2/BCH Decoder  n=47040  k=39200  specShortening=off  shortenedK=5  specGenPoly=off  genPoly='X^10 + X^8 + X^5 + X^4 + X^2 + X + 1'  specPrimPoly=off  prPoly='X^4 + X + 1'  specDisableGenCheck=off  specPuncture=off  punctVec=[ones(8,1); zeros(2,1)]  specErasurePort=off  showNumErr=off
  OFDM Demodulator1 : commofdm/OFDM Demodulator  StatePerturbationForJacobian=1.0e-05  FFTLength=4096  NumGuardBandCarriers=[88; 88]  RemoveDCCarrier=off  PilotOutputPort=off  PilotCarrierIndices=[35;60;85;110;135;160;185;210;235;260;285;310;335;360;385;410;435;460;485;510;535;560;585;610;635;660;685;710;735;760;785;810;835;860;885;910;935;960;985;1010;1035;1060;1085;1110;1135;1160;1185;1210;1235;1260;1285;1310;1335;1360;1385;1410;1435;1460;1485;1510;1535;1560;1585;1610;1635;1660;1685;1710;1735;1760;1785;1810;1835;1860;1885;1910;1935;1960;1985;2010;2035]  CyclicPrefixLength=0  OversamplingFactor=1  NumSymbols=1  NumReceiveAntennas=1  SimulateUsing=Interpreted execution
  Rectangular QAM Demodulator Baseband1 : commdigbbndam3/Rectangular QAM Demodulator Baseband  M=4096  OutType=Bit  DecType=Hard decision  VarSource=Dialog  Variance=1  Dec=Gray  Mapping=[0:15]  PowType=Min. distance between symbols  MinDist=2  AvgPow=1  PeakPow=1  Ph=0  outDtype1=Inherit via internal rule  outDtype2=Inherit via internal rule  derotateFactorWordLen=16  derotateFactorDataTypeStr=Inherit: Same word length as input  derotateFactorLastDataTypeStr=Inherit: Same word length as input  denormFactorWordLen=16  denormFactorDataTypeStr=Inherit: Same word length as input  denormFactorLastDataTypeStr=Inherit: Same word length as input  prodOutWordLen=32  prodOutOverflowMode=Wrap  prodOutRoundingMode=Floor  prodOutOvFlMode=off  prodOutOvFlModeLastStrValue=off  sumWordLen=32
      settings: LibrarySourceBlock=|
      | commhdldigbbndam/Rectangular QAM
      | Demodulator
      | Baseband
  Out1 : Outport
  wires:
  BCH Decoder1/1 -> Out1/1
  OFDM Demodulator1/1 -> Rectangular QAM Demodulator Baseband1/1
  In1/1 -> OFDM Demodulator1/1
  Rectangular QAM Demodulator Baseband1/1 -> BCH Decoder1/1

== system R/Subsystem1/MCS13 WiFi Demodulator24 ==
  In1 : Inport
  BCH Decoder1 : commblkcod2/BCH Decoder  n=47040  k=39200  specShortening=off  shortenedK=5  specGenPoly=off  genPoly='X^10 + X^8 + X^5 + X^4 + X^2 + X + 1'  specPrimPoly=off  prPoly='X^4 + X + 1'  specDisableGenCheck=off  specPuncture=off  punctVec=[ones(8,1); zeros(2,1)]  specErasurePort=off  showNumErr=off
  OFDM Demodulator1 : commofdm/OFDM Demodulator  StatePerturbationForJacobian=1.0e-05  FFTLength=4096  NumGuardBandCarriers=[88; 88]  RemoveDCCarrier=off  PilotOutputPort=off  PilotCarrierIndices=[35;60;85;110;135;160;185;210;235;260;285;310;335;360;385;410;435;460;485;510;535;560;585;610;635;660;685;710;735;760;785;810;835;860;885;910;935;960;985;1010;1035;1060;1085;1110;1135;1160;1185;1210;1235;1260;1285;1310;1335;1360;1385;1410;1435;1460;1485;1510;1535;1560;1585;1610;1635;1660;1685;1710;1735;1760;1785;1810;1835;1860;1885;1910;1935;1960;1985;2010;2035]  CyclicPrefixLength=0  OversamplingFactor=1  NumSymbols=1  NumReceiveAntennas=1  SimulateUsing=Interpreted execution
  Rectangular QAM Demodulator Baseband1 : commdigbbndam3/Rectangular QAM Demodulator Baseband  M=4096  OutType=Bit  DecType=Hard decision  VarSource=Dialog  Variance=1  Dec=Gray  Mapping=[0:15]  PowType=Min. distance between symbols  MinDist=2  AvgPow=1  PeakPow=1  Ph=0  outDtype1=Inherit via internal rule  outDtype2=Inherit via internal rule  derotateFactorWordLen=16  derotateFactorDataTypeStr=Inherit: Same word length as input  derotateFactorLastDataTypeStr=Inherit: Same word length as input  denormFactorWordLen=16  denormFactorDataTypeStr=Inherit: Same word length as input  denormFactorLastDataTypeStr=Inherit: Same word length as input  prodOutWordLen=32  prodOutOverflowMode=Wrap  prodOutRoundingMode=Floor  prodOutOvFlMode=off  prodOutOvFlModeLastStrValue=off  sumWordLen=32
      settings: LibrarySourceBlock=|
      | commhdldigbbndam/Rectangular QAM
      | Demodulator
      | Baseband
  Out1 : Outport
  wires:
  BCH Decoder1/1 -> Out1/1
  OFDM Demodulator1/1 -> Rectangular QAM Demodulator Baseband1/1
  In1/1 -> OFDM Demodulator1/1
  Rectangular QAM Demodulator Baseband1/1 -> BCH Decoder1/1
